simulink library "RgainyBtc"  (R2022b)
settings: Solver=VariableStepAuto  StartTime=0.0  StopTime=10.0  RelTol=1e-3
libraries: HandyTextFile x4, $bdroot x4, AudioStats x2, SetDsm x2
settings Model: Creator=kl13806  LastModifiedBy=kl13806
settings SolverCC: AlgebraicLoopSolver=TrustRegion
settings DebuggingCC: UnconnectedInputMsg=warning  UnconnectedOutputMsg=warning  UnconnectedLineMsg=warning  SFMachineParentedDataDiag=warning
settings ModelReferenceCC: EnableRefExpFcnMdlSchedulingChecks=on
settings RTWCC: DLArmComputeVersion=19.05

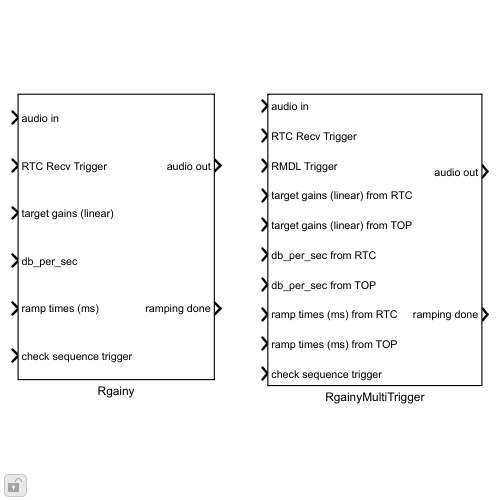
[thumbnail: Simulink's stored preview of the top-level diagram]
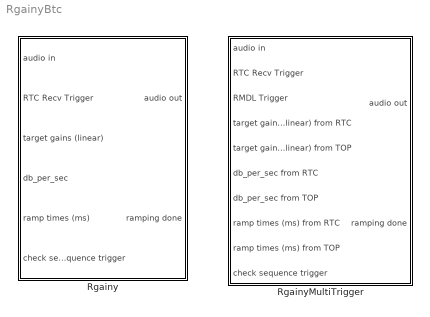
== system RgainyBtc ==
  Rgainy : Subsystem  mask(Blocklib Rgainy){GainOutEnable=off, Config=[]}
      mask prompts: GainOutEnable "Enable Gain Output Port"; Config "RgainyConfig"
      mask help:
      | The RGAINY block can receive an audio input with an arbitary number of channels. The block is instatiated to have a specified number of rampers. The channel-to-ramper map indicates for each channel which ramper number to use or 0 for no ramping. If the ramper map has fewer entries than there are channels, then the last channel's ramper association is repeated for all the unspecified channels.
      |
      | If a non-zero db_per_sec signal is provided, ramp time in milliseconds is ignored. To use time-based ramping, set db_per_sec to zero and use ramp times (either a single time or a vector of times for each ramper will be accepted.)
      |
      | Unlike the BDSP rgainx, this block does not support sharing coefficients among rampers.
      mask init:
      | blkh=gcbh;
      | Config=BTConfig.Assert(blkh,Config);
      | Config.Validate();
      | 
      | % MaskBlockH is passed to an AudioStatsFunc block as a mask parameter.
      | % Simulink block handles (e.g. numeric double) change every time a model
      | % loads - so they would cause the model checksum to also change!
      | % Pass a Simulink block path instead which does not change every time!
      | MaskBlockH = gcb;
      | 
      | RgainyMask.Init(blkh,'gain_out',GainOutEnable);
      mask Help: This block supports either slope-based or time-based control. To use time-based control, ground the db_per_sec input (i.e. sets it to zero) so the ramp_times_ms input will apply. For slope-based control, set the db_per_sec to a non-zero value defining the slope and the ramp_times_ms input will be ignored.
  RgainyMultiTrigger : Subsystem  InitFcn=|  mask(Blocklib RgainyMultiTrigger){GainOutEnable=off, Config=[]}
      | GainLibrary_data
      | RgainName = "Rgainy";
      mask prompts: GainOutEnable "Enable Gain Output Port"; Config "RgainyMultiTriggerConfig"
      mask help:
      | The RGAINY block can receive an audio input with an arbitary number of channels. The block is instatiated to have a specified number of rampers. The channel-to-ramper map indicates for each channel which ramper number to use or 0 for no ramping. If the ramper map has fewer entries than there are channels, then the last channel's ramper association is repeated for all the unspecified channels.
      |
      | If a non-zero db_per_sec signal is provided, ramp time in milliseconds is ignored. To use time-based ramping, set db_per_sec to zero and use ramp times (either a single time or a vector of times for each ramper will be accepted.)
      |
      | Unlike the BDSP rgainx, this block does not support sharing coefficients among rampers.
      mask init:
      | blkh=gcbh;
      | Config=BTConfig.Assert(blkh,Config);
      | Config.Validate();
      |  
      | % MaskBlockH is passed to an AudioStatsFunc block as a mask parameter.
      | % Simulink block handles (e.g. numeric double) change every time a model
      | % loads - so they would cause the model checksum to also change!
      | % Pass a Simulink block path instead which does not change every time!
      | MaskBlockH = gcb;
      | 
      | RgainyMask.Init(blkh,'gain_out',GainOutEnable);
      mask Help: This block supports either slope-based or time-based control. To use time-based control, ground the db_per_sec input (i.e. sets it to zero) so the ramp_times_ms input will apply. For slope-based control, set the db_per_sec to a non-zero value defining the slope and the ramp_times_ms input will be ignored.
      mask Display:
      | % retrieve the block's pixel size
      | pos = get(gcbh,'position');
      | bw = pos(3) - pos(1);
      | bh = pos(4) - pos(2);
      | 
      | % show the message path or a big red X when disabled
      | theMask = Simulink.Mask.get(gcbh);
      | errorText = theMask.getDialogControl('ErrorText');
      | if (false == isempty(errorText) && false == isempty(errorText.Prompt))
      |     tx=bw*0.03;
      |     ty=bh*0.03;
      |     patch([0 tx bw bw-tx], [ty 0 bh-ty bh], [1 0 0]);
      |     patch([0 bw-tx bw tx], [bh-ty 0 ty bh], [1 0 0]);
      | end

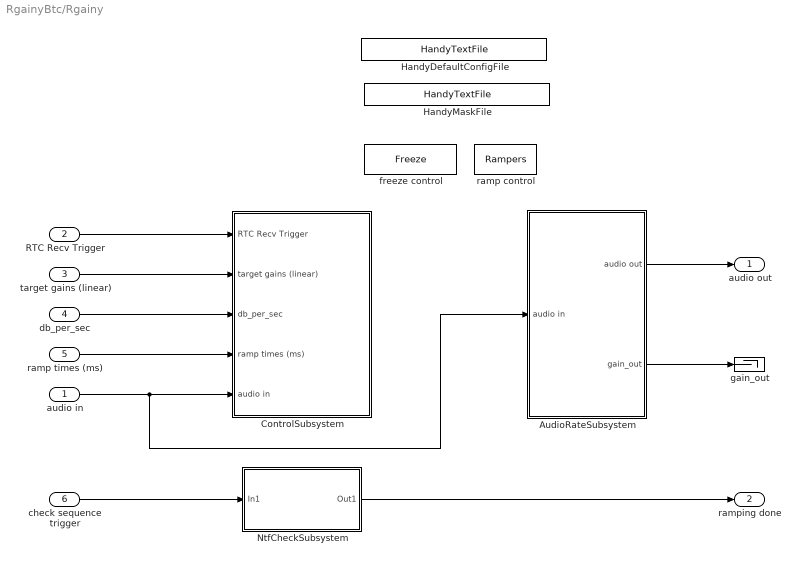
== system RgainyBtc/Rgainy ==
  audio in : Inport
  RTC Recv Trigger : Inport  Port=2
  target gains (linear) : Inport  Port=3
  db_per_sec : Inport  Port=4
  ramp times (ms) : Inport  Port=5
  check sequence trigger : Inport  Port=6
  AudioRateSubsystem : Subsystem
  ControlSubsystem : Subsystem
  HandyDefaultConfigFile : HandyTextFile/HandyTextFile  TemplateSource=Config  FileSuffix=Init  OpenDialogOnLoad=off  UseThisBlockName=off  TheDefaultText=|  ShowInLibBrowser=on
      | % $(FILENAME) Setup model parameters for each "Init" callback (e.g. update diagram)
      | sample_rate_in_hertz = 44100;
      | frame_size = 32;
      | sysin_channel_count = 2;
      settings: SourceProductName=Bose Talaria
  HandyMaskFile : HandyTextFile/HandyTextFile  TemplateSource=Mask  FileSuffix=Init  OpenDialogOnLoad=off  UseThisBlockName=off  TheDefaultText=|  ShowInLibBrowser=on
      | % $(FILENAME) Setup model parameters for each "Init" callback (e.g. update diagram)
      | sample_rate_in_hertz = 44100;
      | frame_size = 32;
      | sysin_channel_count = 2;
      settings: SourceProductName=Bose Talaria
  NtfCheckSubsystem : Subsystem
  freeze control : DataStoreMemory  DataStoreName=Freeze  EmbeddedSignalClassName=Bose.Signal  ShowAdditionalParam=off  OutDataTypeStr=uint32
  gain_out : Terminator
  ramp control : DataStoreMemory  DataStoreName=Rampers  InitialValue=Config.DlgRamperInit  EmbeddedSignalClassName=Bose.Signal  ShowAdditionalParam=off  OutDataTypeStr=Bus: rgain_bus
  audio out : Outport  VectorParamsAs1DForOutWhenUnconnected=off
  ramping done : Outport  Port=2  VectorParamsAs1DForOutWhenUnconnected=off
  wires:
  RTC Recv Trigger/1 -> ControlSubsystem/1(RTC Recv Trigger)
  target gains (linear)/1 -> ControlSubsystem/2(target gains (linear))
  db_per_sec/1 -> ControlSubsystem/3(db_per_sec)
  ramp times (ms)/1 -> ControlSubsystem/4(ramp times (ms))
  audio in/1 -> AudioRateSubsystem/1(audio in), ControlSubsystem/5(audio in)
  AudioRateSubsystem/1(audio out) -> audio out/1
  AudioRateSubsystem/2(gain_out) -> gain_out/1
  check sequence trigger/1 -> NtfCheckSubsystem/1(In1)
  NtfCheckSubsystem/1(Out1) -> ramping done/1

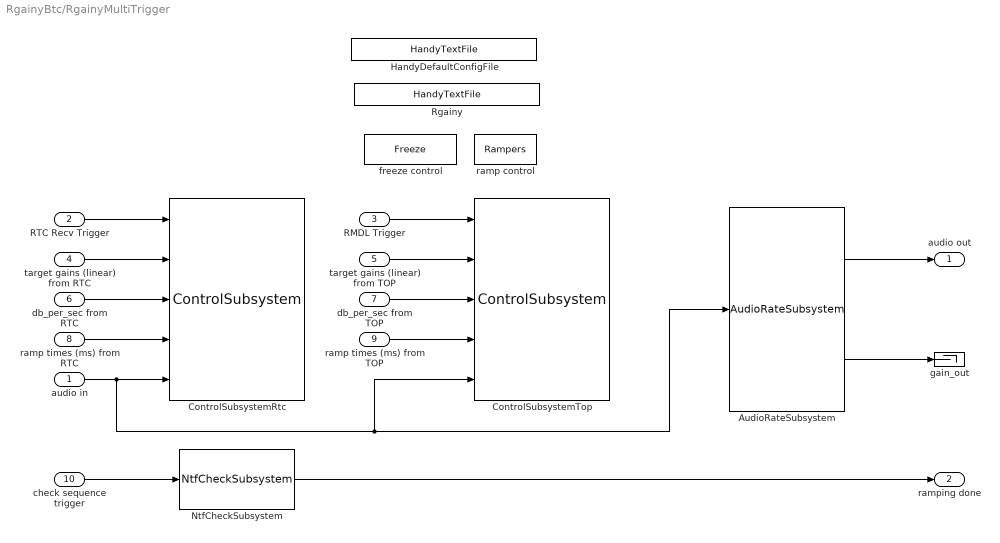
== system RgainyBtc/RgainyMultiTrigger ==
  audio in : Inport
  RTC Recv Trigger : Inport  Port=2
  RMDL Trigger : Inport  Port=3
  target gains (linear) from RTC : Inport  Port=4
  target gains (linear) from TOP : Inport  Port=5
  db_per_sec from RTC : Inport  Port=6
  db_per_sec from TOP : Inport  Port=7
  ramp times (ms) from RTC : Inport  Port=8
  ramp times (ms) from TOP : Inport  Port=9
  check sequence trigger : Inport  Port=10
  AudioRateSubsystem : $bdroot/Rgainy/AudioRateSubsystem  SystemSampleTime=-1  VariantActivationTime=update diagram  Latency=0  AutoFrameSizeCalculation=off
  ControlSubsystemRtc : $bdroot/Rgainy/ControlSubsystem  SystemSampleTime=-1  VariantActivationTime=update diagram  Latency=0  AutoFrameSizeCalculation=off
  ControlSubsystemTop : $bdroot/Rgainy/ControlSubsystem  SystemSampleTime=-1  VariantActivationTime=update diagram  Latency=0  AutoFrameSizeCalculation=off
  HandyDefaultConfigFile : HandyTextFile/HandyTextFile  TemplateSource=Config  FileSuffix=Init  OpenDialogOnLoad=off  UseThisBlockName=off  TheDefaultText=|  ShowInLibBrowser=on
      | % $(FILENAME) Setup model parameters for each "Init" callback (e.g. update diagram)
      | sample_rate_in_hertz = 44100;
      | frame_size = 32;
      | sysin_channel_count = 2;
      settings: SourceProductName=Bose Talaria
  NtfCheckSubsystem : $bdroot/Rgainy/NtfCheckSubsystem  SystemSampleTime=-1  VariantActivationTime=update diagram  Latency=0  AutoFrameSizeCalculation=off
  Rgainy : HandyTextFile/HandyTextFile  TemplateSource=Mask  FileSuffix=Init  OpenDialogOnLoad=off  UseThisBlockName=on  TheDefaultText=|  ShowInLibBrowser=on
      | % $(FILENAME) Setup model parameters for each "Init" callback (e.g. update diagram)
      | sample_rate_in_hertz = 44100;
      | frame_size = 32;
      | sysin_channel_count = 2;
      settings: SourceProductName=Bose Talaria
  freeze control : DataStoreMemory  DataStoreName=Freeze  EmbeddedSignalClassName=Bose.Signal  ShowAdditionalParam=off  OutDataTypeStr=uint32
  gain_out : Terminator
  ramp control : DataStoreMemory  DataStoreName=Rampers  InitialValue=Config.DlgRamperInit  EmbeddedSignalClassName=Bose.Signal  ShowAdditionalParam=off  OutDataTypeStr=Bus: rgain_bus
  audio out : Outport  VectorParamsAs1DForOutWhenUnconnected=off
  ramping done : Outport  Port=2  VectorParamsAs1DForOutWhenUnconnected=off
  wires:
  AudioRateSubsystem/2 -> gain_out/1
  AudioRateSubsystem/1 -> audio out/1
  RTC Recv Trigger/1 -> ControlSubsystemRtc/1
  target gains (linear) from RTC/1 -> ControlSubsystemRtc/2
  db_per_sec from RTC/1 -> ControlSubsystemRtc/3
  ramp times (ms) from RTC/1 -> ControlSubsystemRtc/4
  audio in/1 -> AudioRateSubsystem/1, ControlSubsystemTop/5, ControlSubsystemRtc/5
  RMDL Trigger/1 -> ControlSubsystemTop/1
  target gains (linear) from TOP/1 -> ControlSubsystemTop/2
  db_per_sec from TOP/1 -> ControlSubsystemTop/3
  ramp times (ms) from TOP/1 -> ControlSubsystemTop/4
  check sequence trigger/1 -> NtfCheckSubsystem/1
  NtfCheckSubsystem/1 -> ramping done/1

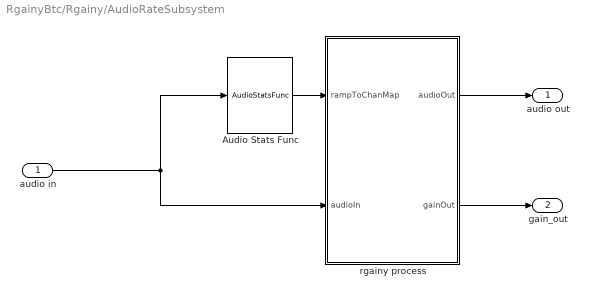
== system RgainyBtc/Rgainy/AudioRateSubsystem ==
  audio in : Inport
  Audio Stats Func : AudioStats/AudioStatsFunc  UserFuncName=RgainyMask.ConvertChan2RampIntoRamp2Chan  Do1=off  Type1=single  Do2=off  Type2=single  Do3=on  Type3=single  AdditionalInArgs=MaskBlockH,Config  TriggerInit=[225 42 290 118]  MaskOutNames=map
      settings: SourceProductName=Bose Talaria
  rgainy process : MATLAB Function  TreatAsAtomicUnit=on  mask{MaskNumRampers=Config.NumRampers}
  audio out : Outport  VectorParamsAs1DForOutWhenUnconnected=off
  gain_out : Outport  Port=2
  wires:
  audio in/1 -> rgainy process/2(audioIn), Audio Stats Func/1
  rgainy process/1(audioOut) -> audio out/1
  Audio Stats Func/1 -> rgainy process/1(rampToChanMap)
  rgainy process/2(gainOut) -> gain_out/1

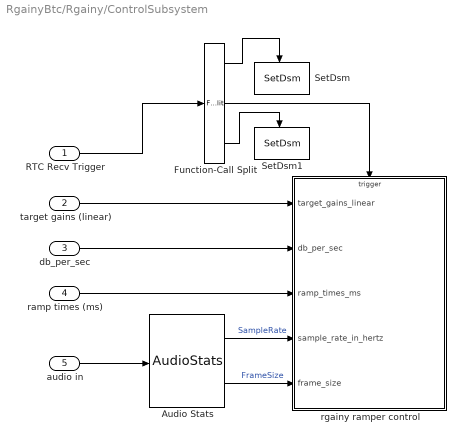
== system RgainyBtc/Rgainy/ControlSubsystem ==
  RTC Recv Trigger : Inport
  target gains (linear) : Inport  Port=2
  db_per_sec : Inport  Port=3
  ramp times (ms) : Inport  Port=4
  audio in : Inport  Port=5
  Audio Stats : AudioStats/AudioStats  DoSampleRate=on  TypeSampleRate=Inherit: auto  DoCallRate=off  TypeCallRate=Inherit: auto  DoFrameSize=on  TypeFrameSize=Inherit: auto  DoChannelCount=off  TypeChannelCount=Inherit: auto  DoTaskRateFactor=off  TypeTaskRateFactor=Inherit: auto  MacroNameRoot=AUDIO  MacroNameRootEval='AUDIO'  IsMacroNameEval=off  MacroSampleRate=off  MacroCallRate=off  MacroFrameSize=off  MacroChannelCount=off  MacroTaskRateFactor=off  MacroTaskId=off  ValidateSampleRate=off  ValueSampleRate=44100  ValidateCallRate=off  ValueCallRate=[]  ValidateFrameSize=off  ValueFrameSize=32  ValidateChannelCount=off  ValueChannelCount=[]  ValidateTaskRateFactor=off  ValueTaskRateFactor=[]
      settings: SourceProductName=Bose Talaria
  Function-Call Split : FunctionCallSplit  IconShape=distinctive  NumOutputPorts=3  OutputPortLayout=default
  SetDsm : SetDsm/SetDsm  DataStoreName=Freeze  Value=uint32(1)
      settings: SourceProductName=Bose Talaria
  SetDsm1 : SetDsm/SetDsm  DataStoreName=Freeze  Value=uint32(0)
      settings: SourceProductName=Bose Talaria
  rgainy ramper control : MATLAB Function  TreatAsAtomicUnit=on  mask{MaskNumRampers=Config.NumRampers}
  wires:
  Audio Stats/1 -> rgainy ramper control/4(sample_rate_in_hertz)  "SampleRate"
  target gains (linear)/1 -> rgainy ramper control/1(target_gains_linear)
  audio in/1 -> Audio Stats/1
  db_per_sec/1 -> rgainy ramper control/2(db_per_sec)
  ramp times (ms)/1 -> rgainy ramper control/3(ramp_times_ms)
  RTC Recv Trigger/1 -> Function-Call Split/1
  Audio Stats/2 -> rgainy ramper control/5(frame_size)  "FrameSize"
  Function-Call Split/1 -> SetDsm/Trigger
  Function-Call Split/2 -> rgainy ramper control/Trigger
  Function-Call Split/3 -> SetDsm1/Trigger

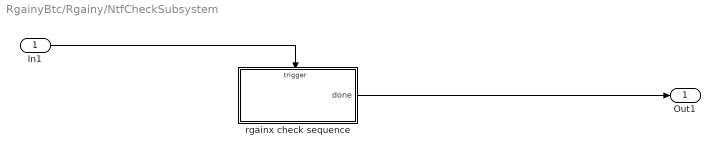
== system RgainyBtc/Rgainy/NtfCheckSubsystem ==
  In1 : Inport
  rgainx check sequence : MATLAB Function  TreatAsAtomicUnit=on  mask{MaskNumRampers=Config.NumRampers}
  Out1 : Outport
  wires:
  In1/1 -> rgainx check sequence/Trigger
  rgainx check sequence/1(done) -> Out1/1

== matlab function RgainyBtc/Rgainy/ControlSubsystem/rgainy ramper control ==
  data target_gains_linear settings: description=This vector signal must provide a linear target gain for every ramper.
  data db_per_sec settings: description="If provided (i.e. non zero), this argument causes the \"ramp times (ms)\" input to be ignored. The block will calculate ramp times itself to ensure all gain changes happen at the db_per_sec slope provided."
  data ramp_times_ms settings: description=|
      | The rampTimes_ms signal can accept one or more ramp times. If only one time is given, it is applied to all rampers. When more than one time is given, the times are delt out to the rampers in order. If not enough times are specified to cover all the rampers, the last given time is filled in to any remaining rampers.
      | NOTE: this input signal is entirely ignored if the db_per_sec input signal is non-zero. Attach the db_per_sec input to a ground block if you want to provide ramp times via this input.
  data sample_rate_in_hertz settings: description="This input is required for control calculations to work. The \"Audio Stats\" block is a handy tool to lift this property right off an inbound audio signal and feed it to this block automatically without using workspace parameters or other constants."
  data frame_size settings: description="This input is required for control calculations to work. The \"Audio Stats\" block is a handy tool to lift this property right off an inbound audio signal and feed it to this block automatically without using workspace parameters or other constants."
  data: target_gains_linear input size=[1 MaskNumRampers]; db_per_sec input; ramp_times_ms input; sample_rate_in_hertz input; frame_size input; Rampers data_store_memory; MaskNumRampers parameter
  events: trigger input FUNCTION_CALL_EVENT
function control(...
     target_gains_linear, db_per_sec, ramp_times_ms, sample_rate_in_hertz, ...
     frame_size, MaskNumRampers)
%#codegen

% Dimensions of target_gains_linear must match the number of rampers. 
%
% db_per_sec takes precidence:
% If db_per_sec has a non-zero value then any ramp_times_ms values are
% ignored and the db_per_sec is used to determine ramper timing.
%
% The dimension of ramp_times_ms is flexible and does not need to match the
% ramper count. Its values are assigned to rampers in rotating order. If
% there are 5 rampers and only two times provided, then rampers 1,3, and 5
% get the first ramp time and rampers 2 and 4 receive the second ramp time.
% Any extra ramp times (beyond the number of rampers) are silently ignored.

global Rampers;

rgain_SILENT_GAIN = RgainBusUtil.GetSilentGainLinear();

% Get the sizes of the provided target and time specifications
numGains = numel(target_gains_linear);
numTimes = numel(ramp_times_ms);
numdbpersecs=numel(db_per_sec);

% Step 1: FREEZE the gain ramper so that we can perform calculations based
% on the current gain value. (This step is done outside on canvas now)

for ramper=1:MaskNumRampers
    
    % assign gains and ramp times
    targetGain = single(target_gains_linear(mod(ramper-1,numGains)+1));
    ramp_ms    = single(ramp_times_ms      (mod(ramper-1,numTimes)+1));
    ramp_dbPerSec= single(db_per_sec      (mod(ramper-1,numdbpersecs)+1));

    % Step 2: Nudge the gain values a bit if they are sitting at zero.
    % When this control set goes live, ensure that the current gain will move.
    % If current gain is zero, replace with a value very close to zero. What we
    % really want is a value which is on the edge of perception - not too small
    % or large. If the value is too small, we'll waste some of our ramp time
    % in perceived silence. If the value is too large, the audio will lurch
    % into perceptability at the start of the ramp.
    currentGain = max(Rampers(ramper).currentGain, rgain_SILENT_GAIN);
    targetGain  = max(targetGain, rgain_SILENT_GAIN);
    
    % Step 3a: If a slope in dB/second is provided, ignore the ramp time
    % and instead calculate a new ramp time that matches the slope.
    if (ramp_dbPerSec)
        currentGain_db = 20*log10(currentGain);
        targetGain_db = 20*log10(targetGain);
        diff = abs(currentGain_db - targetGain_db);
        ramp_ms = diff / single(ramp_dbPerSec) * 1000;
    end
    
    % Step 3b: QUANTIZE the desired ramp time to our FrameSize. Also retrieve 
    % the whole number of frames required to best match requested ramp time.
    % Ensure that at least one frame is used. The frame size will therefore
    % determine the steepest ramp (i.e. within one frame you can go anywhere).
    quantum_ms = 1000 * frame_size / sample_rate_in_hertz;
    numFrames = ramp_ms / quantum_ms;
    % Do a ceil rather than a round to insure that we create enough
    % frames. i.e. a fraction of a frame is promoted to an addition frame
    % numFrames = max (1, round(numFrames));
    numFrames = max (1, ceil(numFrames));
    quantized_rampTime_ms = numFrames * quantum_ms;
   
    % In order to have the desired ramp time, the slope must vary dependent
    % on the gain differencebetween target and current value.
    % Ramper's coefficient is therefore calculated as follows:
    %
    %   TargetGain = CurrentGain *( RampCoef ^ (Fs*RampTime_ms/1000) )
    %
    % therefore...
    %
    %                     log(TargetGain/CurrentGain)
    %   log(RampCoef) = ------------------------------
    %                        Fs*(RampTime_ms/1000)
    %
    factor = log( targetGain / currentGain );
    RampCoef = exp(factor / (sample_rate_in_hertz * quantized_rampTime_ms / 1000));

    % Output control signals
    Rampers(ramper).frameCount  = int32(numFrames);
    Rampers(ramper).rampCoeff   = single(RampCoef);
    Rampers(ramper).targetGain  = target_gains_linear(ramper);
    Rampers(ramper).currentGain = currentGain;
end
% Step 4: UNFREEZE the gain ramper (performed outside on canvas now)

== matlab function RgainyBtc/Rgainy/NtfCheckSubsystem/rgainx check sequence ==
  data: done output; Rampers data_store_memory; MaskNumRampers parameter
  events: trigger input FUNCTION_CALL_EVENT
function done = GetCompletedSequence(MaskNumRampers)
% Check if the ramping is done by comparing the target and current gains.

global Rampers;

% Assume the work is complete until proven otherwise
done = true;
for i=1:MaskNumRampers
   if (Rampers(i).targetGain ~= Rampers(i).currentGain)
       done = false; % just proved otherwise
       break;
   end
end

== matlab function RgainyBtc/Rgainy/AudioRateSubsystem/rgainy process ==
  data: rampToChanMap input; audioIn input; audioOut output; Rampers data_store_memory; Freeze data_store_memory; MaskNumRampers parameter; gainOut output
function [audioOut, gainOut]  = rgainx(rampToChanMap, audioIn, MaskNumRampers)
%#codegen

global Rampers;
global Freeze;

% set the size of the output buffer
audioOut = coder.nullcopy(audioIn);

[frame_size,channel_count] = size(audioIn);
gainOut = single(ones(1,channel_count));

% Channel indexes start in the map just after the ramper channel counts.
% Create an iterator to walk the channel indexes in rampToChanMap
% (set its value to "point" just *before* the first channel index, since
% we'll add a channel count to it during use below)
chanIterator = cast(MaskNumRampers,'like',rampToChanMap);

% Loop through rampers and apply their gain coefficients
for ramper = 1:MaskNumRampers
    k = single(1);
    gain = Rampers(ramper).currentGain;
    if (Freeze(1) == false)
        if (Rampers(ramper).frameCount == 0)
            % The ramp is finished. Stop ramping and SNAP to the target
             gain = Rampers(ramper).targetGain;
        else
            % The ramp is *NOT* frozen or done: gain is moving
            k = Rampers(ramper).rampCoeff;
            Rampers(ramper).frameCount = Rampers(ramper).frameCount - 1;
        end
    end
    % Loop through samples, adjusting gain and applying to channels
    for n=1:frame_size
        gain = gain * k;
        % Loop through channels associated with this ramper
        for chanCount = 1:rampToChanMap(ramper)
            chanIdx = rampToChanMap(chanIterator + chanCount);
            audioOut(n,chanIdx) = audioIn(n,chanIdx) * gain;
        end
    end
    for chanCount = 1:rampToChanMap(ramper)
        chanIdx = rampToChanMap(chanIterator + chanCount);
        gainOut(chanIdx) = gain;
    end
    Rampers(ramper).currentGain = gain;
    chanIterator = chanIterator + rampToChanMap(ramper);
end
% handle any channels that are not assigned to a ramper (i.e. no gain)
for noRampChannel=(chanIterator+1):(channel_count+MaskNumRampers)
    chanIdx = rampToChanMap(noRampChannel);
    for n=1:frame_size
            audioOut(n,chanIdx) = audioIn(n,chanIdx);
    end
end
